simulink model "MAVmodel"  (R2016a)
settings: Solver=VariableStepAuto  StartTime=0.0  StopTime=10.0  RelTol=1e-3
libraries: aerolib6dof2 x1
settings Model: Creator=Giliam  LastModifiedBy=Giliam

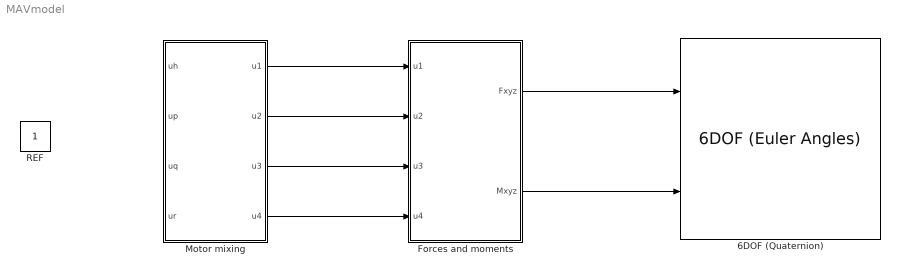
== system MAVmodel ==
  6DOF (Quaternion) : aerolib6dof2/6DOF (Euler Angles)  units=Metric (MKS)  mtype=Fixed  rep=Quaternion  xme_0=[0 0 0]  Vm_0=[0 0 0]  eul_0=[0 0 0]  pm_0=[0 0 0]  mass_0=1.0  mass_e=0.5  mass_f=2.0  inertia=eye(3)  inertia_e=eye(3)  inertia_f=2*eye(3)  k_quat=1.0  vre_flag=on
  Forces and moments : Subsystem
  Motor mixing : Subsystem
  REF : Constant
  wires:
  Motor mixing/1(u1) -> Forces and moments/1(u1)
  Motor mixing/2(u2) -> Forces and moments/2(u2)
  Motor mixing/3(u3) -> Forces and moments/3(u3)
  Motor mixing/4(u4) -> Forces and moments/4(u4)
  Forces and moments/1(Fxyz) -> 6DOF (Quaternion)/1
  Forces and moments/2(Mxyz) -> 6DOF (Quaternion)/2

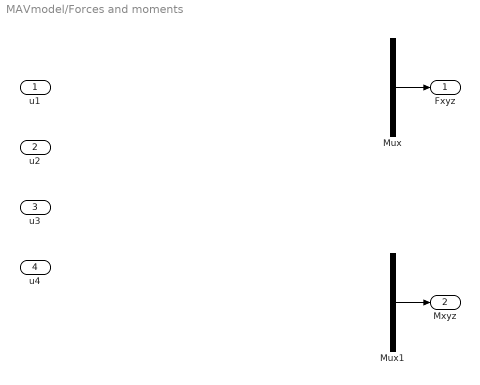
== system MAVmodel/Forces and moments ==
  u1 : Inport
  u2 : Inport  Port=2
  u3 : Inport  Port=3
  u4 : Inport  Port=4
  Mux : Mux  Inputs=3
  Mux1 : Mux  Inputs=3
  Fxyz : Outport
  Mxyz : Outport  Port=2
  wires:
  Mux/1 -> Fxyz/1
  Mux1/1 -> Mxyz/1

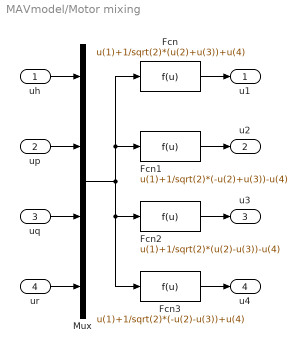
== system MAVmodel/Motor mixing ==
  uh : Inport
  up : Inport  Port=2
  uq : Inport  Port=3
  ur : Inport  Port=4
  Fcn : Fcn  Expr=u(1)+1/sqrt(2)*(u(2)+u(3))+u(4)
  Fcn1 : Fcn  Expr=u(1)+1/sqrt(2)*(-u(2)+u(3))-u(4)
  Fcn2 : Fcn  Expr=u(1)+1/sqrt(2)*(u(2)-u(3))-u(4)
  Fcn3 : Fcn  Expr=u(1)+1/sqrt(2)*(-u(2)-u(3))+u(4)
  Mux : Mux
  u1 : Outport
  u2 : Outport  Port=2
  u3 : Outport  Port=3
  u4 : Outport  Port=4
  wires:
  uh/1 -> Mux/1
  up/1 -> Mux/2
  uq/1 -> Mux/3
  ur/1 -> Mux/4
  Mux/1 -> Fcn3/1, Fcn2/1, Fcn1/1, Fcn/1
  Fcn3/1 -> u4/1
  Fcn2/1 -> u3/1
  Fcn1/1 -> u2/1
  Fcn/1 -> u1/1
